simulink model "HF"  (Simulink 10.0)
settings: Solver=ode3  StartTime=0.0  StopTime=8  FixedStep=Tsim  RelTol=1e-3  EnableMultiTasking=on
InitFcn:
  | Tsim=2e-7;
values from neighbouring files (symbols this model uses):
  Flux = 0.00529276    [Hall_HFI_FOC_Data.sldd]
undefined symbols (not defined in the file or in its folder): DiscIntNeverNeededParam, sigbuilder_block
libraries: powerlib x10, powerlib_meascontrol x4, powerlib_extras x1, simulink_extras x1
settings Model: Creator=Administrator  LastModifiedBy=Administrator  SimulationMode=accelerator
settings DataIOCC: LimitDataPoints=on  SaveFormat=StructureWithTime
settings OptimizationCC: EfficientMapNaN2IntZero=off
settings DebuggingCC: UnderspecifiedInitializationDetection=Simplified  MergeDetectMultiDrivingBlocksExec=error
settings HardwareCC: ProdBitPerPointer=64  ProdLargestAtomicFloat=Float  ProdIntDivRoundTo=Zero  ProdEndianess=LittleEndian  ProdHWDeviceType=Specified  TargetBitPerPointer=64  TargetBitPerSizeT=64  TargetBitPerPtrDiffT=64  TargetLongLongMode=on  TargetIntDivRoundTo=Zero  TargetEndianess=LittleEndian  TargetWordSize=64  TargetHWDeviceType=MATLAB Host  ProdEqTarget=off
settings CodeAppCC: MaxIdLength=128
settings GRTTargetCC: GeneratePreprocessorConditionals=Disable all
settings ConfigComp: CovExternalEMLEnable=off
settings SimscapeCC: SimscapeNormalizeSystem=off

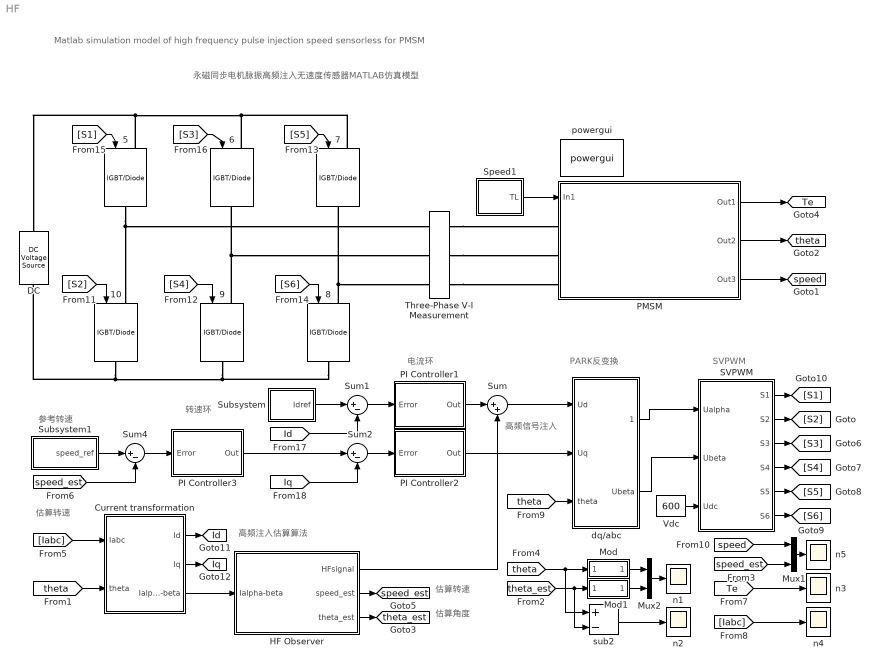
== system HF ==
  note: 转速环
  note: 永磁同步电机脉振高频注入无速度传感器MATLAB仿真模型
  note: Matlab simulation model of high frequency pulse injection speed sensorless for PMSM
  note: 电流环
  note: PARK反变换
  note: SVPWM
  note: 参考转速
  note: 估算转速
  note: 高频信号注入
  note: 估算转速
  note: 估算角度
  note: 高频注入估算算法
  {5..10} (6 alike) : powerlib/Power Electronics/IGBT//Diode  Ron=1e-3  Rs=5000  Cs=inf  Measurements=off
      settings: SourceProductName=Simscape Electrical
  Current transformation : Subsystem
  "DC " : powerlib/Electrical Sources/DC Voltage Source  Amplitude=600  Measurements=None
      settings: SourceProductName=Simscape Electrical
  HF Observer : Subsystem
  Mod : Subsystem
  Mod1 : Subsystem
  Mux1 : Mux  Inputs=2
  Mux2 : Mux  Inputs=2
  PI Controller1 : Subsystem  DialogController=POWERSYS.PowerSysDialog  mask(Discrete PI Controller){Kp=19.8, Ki=4550, Par_Limits=[346.4 -346.4], Init=0, Ts=1e-4}
      mask prompts: Kp "Proportional gain (Kp):"; Ki "Integral gain (Ki):"; Par_Limits "Output limits: [ Upper   Lower ]"; Init "Output initial value:"; Ts "Sample time:"
      mask help: This block implements a discrete PI controller.
      mask init:
      | UpperLimit=Par_Limits(1);
      | LowerLimit=Par_Limits(2);
      | power_initmask();
      mask Help: This block is part of a subset of blocks in the Extras library that does not have documentation associated with it, other than the block mask description.
      mask Display: disp('PI');
  PI Controller2 : Subsystem  DialogController=POWERSYS.PowerSysDialog  mask(Discrete PI Controller){Kp=19.9, Ki=4550, Par_Limits=[346.4 -346.4], Init=0, Ts=1e-4}
      mask prompts: Kp "Proportional gain (Kp):"; Ki "Integral gain (Ki):"; Par_Limits "Output limits: [ Upper   Lower ]"; Init "Output initial value:"; Ts "Sample time:"
      mask help: This block implements a discrete PI controller.
      mask init:
      | UpperLimit=Par_Limits(1);
      | LowerLimit=Par_Limits(2);
      | power_initmask();
      mask Help: This block is part of a subset of blocks in the Extras library that does not have documentation associated with it, other than the block mask description.
      mask Display: disp('PI');
  PI Controller3 : Subsystem  DialogController=POWERSYS.PowerSysDialog  mask(Discrete PI Controller){Kp=5, Ki=60, Par_Limits=[10 -10], Init=0, Ts=1e-4}
      mask prompts: Kp "Proportional gain (Kp):"; Ki "Integral gain (Ki):"; Par_Limits "Output limits: [ Upper   Lower ]"; Init "Output initial value:"; Ts "Sample time:"
      mask help: This block implements a discrete PI controller.
      mask init:
      | UpperLimit=Par_Limits(1);
      | LowerLimit=Par_Limits(2);
      | power_initmask();
      mask Help: This block is part of a subset of blocks in the Extras library that does not have documentation associated with it, other than the block mask description.
      mask Display: disp('PI');
  PMSM : Subsystem
      mask Display: image('PMSM.jpg');
  SVPWM : Subsystem  mask(Seven - sects SVPWM generator){fpwm=10e3, Ts=2e-7}
      mask prompts: fpwm "PWM frequency fpwm (Hz):"; Ts "Sample time Ts (s):"
      mask help: This block implements a space vector PWM.
  Speed1 : Subsystem  Tag=STV Subsys  LoadFcn=sigbuilder_block('load');  StartFcn=sigbuilder_block('start');  StopFcn=sigbuilder_block('stop');  ClipboardFcn=sigbuilder_block('clipboard');  mask(Sigbuilder block){tuvar=[0:10]}
      mask help: Simulink:masks:SigbuilderBlock_MD
      mask init:
      | if ~strcmp(get_param(bdroot(gcbh),'SimulationStatus'),'stopped') tuvar = sigbuilder_block('maskInit'); end
      settings: CopyFcn=sigbuilder_block('copy');  DeleteFcn=sigbuilder_block('delete');  ModelCloseFcn=sigbuilder_block('modelClose');  PreSaveFcn=sigbuilder_block('preSave');  PauseFcn=sigbuilder_block('pause');  ContinueFcn=sigbuilder_block('continue');  NameChangeFcn=sigbuilder_block('namechange');  OpenFcn=sigbuilder_block('open',[6 21.75 1012.5 490.5 ]);  CloseFcn=sigbuilder_block('close');
      mask Display: plot(0, 0, 100, 100,[2, 2, 32, 32, 2], [68, 8, 8, 68, 68],[32, 2], [38, 38], [32, 19, 2],[53, 60, 44], [32, 17, 17, 2],[16, 16, 31, 31]);txt = getActiveGroup(gcbh);text(2, 100, txt,'verticalAlignment', 'top');
  Subsystem : Subsystem
  Subsystem1 : Subsystem
  Sum : Sum  Inputs=|++
  Sum1 : Sum  Inputs=|+-
  Sum2 : Sum  Inputs=|+-
  Sum4 : Sum  Inputs=|+-
  Three-Phase V-I Measurement : powerlib/Measurements/Three-Phase V-I Measurement  VoltageMeasurement=phase-to-phase  SetLabelV=on  LabelV=Vabc  Vpu=off  VpuLL=off  CurrentMeasurement=yes  SetLabelI=on  LabelI=Iabc  Ipu=off  Pbase=100e6  Vbase=500e3  OutputType=Complex  PhasorSimulation=off  PSBequivalent=0
      settings: SourceProductName=Simscape Electrical
  Vdc : Constant  Value=600
  dq/abc : Subsystem
  n{1..5} (5 alike) : Scope
  powergui : powerlib/powergui  Priority=1  SimulationMode=Discrete  SampleTime=0.002*1e-4  frequency=60  Iterations=50  frequencyindice=0  Pbase=100e6  ErrMax=1e-4  UnitsV=kV  UnitsW=MW  buscounter=0  FunctionMessages=off  echomessages=off  EnableUseOfTLC=off  CurrentSourceSwitches=off  DisableSnubberDevices=off  DisableRonSwitches=off  DisableVfSwitches=off  DisplayEquations=off  AutomaticDiscreteSolvers=off  SolverType=Tustin/Backward Euler (TBE)  Interpol=off  ExternalGateDelay=off  methode=off  Ts=10  x0status=blocks  SPID=off  SwTol=0  HookPort=off  NonlinearTolerance=1e-4  nMaxIteration=100  ContinueOnMaxIteration=off  RestoreLinks=warning  ResistiveCurrentMeasurement=off  Frange=[0:2:500]  Ylog=off  Xlog=on  ShowGrid=off  save=off  variable=ZData  structure=0  ZoomFFT=off  StartTime=0.0  cycles=1  DisplayStyle=1  fundamental=60  FreqAxis=off  MaxFrequency=1000  frequencyindicesteady=1  RmsSteady=1  display=off
      settings: SourceProductName=Simscape Electrical
  sub2 : Sum  Inputs=+-
  tag scope: Id=global, Iq=global, Te=global, speed=global, speed_est=global, theta=global, theta_est=global
  wires:
  dq/abc/1(Ualpha) -> SVPWM/1(Ualpha)
  PI Controller3/1(Out) -> Sum2/1
  HF Observer/3(theta_est) -> [theta_est]
  HF Observer/1(HFsignal) -> Sum/2
  PI Controller1/1(Out) -> Sum/1
  Vdc/1 -> SVPWM/3(Udc)
  Sum1/1 -> PI Controller1/1(Error)
  Sum2/1 -> PI Controller2/1(Error)
  Sum4/1 -> PI Controller3/1(Error)
  Mux2/1 -> n1/1
  Mod/1(Out1) -> Mux2/1
  Mod1/1(Out1) -> Mux2/2
  [theta] -> Current transformation/2(theta)
  [theta] -> dq/abc/3(theta)
  [theta_est] -> sub2/2, Mod1/1(In1)
  [theta] -> sub2/1, Mod/1(In1)
  sub2/1 -> n2/1
  PI Controller2/1(Out) -> dq/abc/2(Uq)
  Sum/1 -> dq/abc/1(Ud)
  dq/abc/2(Ubeta) -> SVPWM/2(Ubeta)
  [S1] -> 5/1
  [S2] -> 10/1
  [S3] -> 6/1
  [S4] -> 9/1
  [S5] -> 7/1
  [S6] -> 8/1
  SVPWM/1(S1) -> [S1]
  SVPWM/2(S2) -> [S2]
  SVPWM/3(S3) -> [S3]
  SVPWM/4(S4) -> [S4]
  SVPWM/5(S5) -> [S5]
  SVPWM/6(S6) -> [S6]
  [Iabc] -> Current transformation/1(Iabc)
  Speed1/1(TL) -> PMSM/1(In1)
  PMSM/1(Out1) -> [Te]
  PMSM/2(Out2) -> [theta]
  PMSM/3(Out3) -> [speed]
  [Te] -> n3/1
  [Iabc] -> n4/1
  Current transformation/3(Ialpha-beta) -> HF Observer/1(Ialpha-beta)
  HF Observer/2(speed_est) -> [speed_est]
  [speed_est] -> Sum4/2
  Mux1/1 -> n5/1
  [speed_est] -> Mux1/2
  [speed] -> Mux1/1
  Current transformation/1(Id) -> [Id]
  Current transformation/2(Iq) -> [Iq]
  [Id] -> Sum1/2
  [Iq] -> Sum2/2
  Subsystem1/1(speed_ref) -> Sum4/1
  Subsystem/1(Idref) -> Sum1/1
  connections:
  10/RConn1 -- "DC "/LConn1 -- 8/RConn1 -- 9/RConn1
  5/RConn1 -- Three-Phase V-I Measurement/LConn1 -- 10/LConn1
  9/LConn1 -- Three-Phase V-I Measurement/LConn2 -- 6/RConn1
  8/LConn1 -- Three-Phase V-I Measurement/LConn3 -- 7/RConn1
  5/LConn1 -- "DC "/RConn1 -- 6/LConn1 -- 7/LConn1
  Three-Phase V-I Measurement/RConn1 -- PMSM/LConn1
  Three-Phase V-I Measurement/RConn2 -- PMSM/LConn2
  Three-Phase V-I Measurement/RConn3 -- PMSM/LConn3

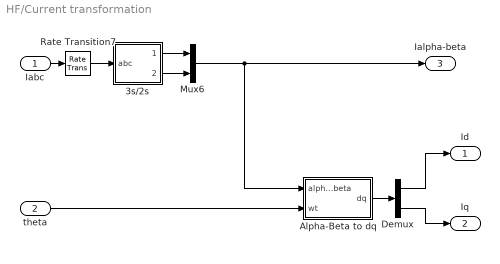
== system HF/Current transformation ==
  Iabc : Inport
  theta : Inport  Port=2
  3s/2s : Subsystem
  Alpha-Beta to dq : Subsystem
      mask Display:
      | plot([0 1], [0,1])
      | port_label('input', 1, '\alpha\beta','texmode','on')
      | port_label('input', 2, 'wt')
      | port_label('output', 1, 'dq')
  Demux : Demux  Outputs=2
  Mux6 : Mux  Inputs=2
  Rate Transition7 : RateTransition
  Id : Outport
  Iq : Outport  Port=2
  Ialpha-beta : Outport  Port=3
  wires:
  Iabc/1 -> Rate Transition7/1
  3s/2s/1(alpha) -> Mux6/1
  3s/2s/2(beta) -> Mux6/2
  Mux6/1 -> Ialpha-beta/1, Alpha-Beta to dq/1(alpha_beta)
  theta/1 -> Alpha-Beta to dq/2(wt)
  Alpha-Beta to dq/1(dq) -> Demux/1
  Demux/1 -> Id/1
  Demux/2 -> Iq/1
  Rate Transition7/1 -> 3s/2s/1(abc)

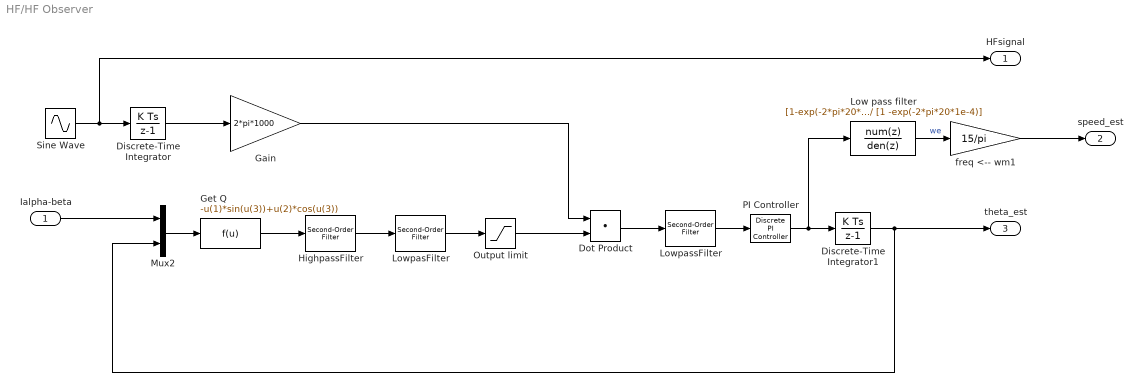
== system HF/HF Observer ==
  Ialpha-beta : Inport
  Discrete-Time Integrator : DiscreteIntegrator  SampleTime=-1  ICPrevOutput=DiscIntNeverNeededParam  ICPrevScaledInput=DiscIntNeverNeededParam
  Discrete-Time Integrator1 : DiscreteIntegrator  SampleTime=-1  ICPrevOutput=DiscIntNeverNeededParam  ICPrevScaledInput=DiscIntNeverNeededParam
  Dot Product : DotProduct  InputSameDT=on  OutDataTypeStr=Inherit: Inherit via internal rule
  Gain : Gain  Gain=2*pi*1000
  Get Q : Fcn  Expr=-u(1)*sin(u(3))+u(2)*cos(u(3))
  HighpassFilter : powerlib_meascontrol/Filters/Second-Order Filter  FilterType=Highpass  Fo=1000 - 100/2  Zeta=0.3  Ts=1e-4  Initialize=off  Vac_Init="[0,  0,  60]"  Vdc_Init=0  PlotResponse=off  FreqRange=[0, 10000, 1]
      settings: SourceProductName=Simscape Electrical  SourceProductBaseCode=PS
  Low pass filter : DiscreteTransferFcn  Numerator=[1-exp(-2*pi*20*1e-4)]  Denominator=[1 -exp(-2*pi*20*1e-4)]  SampleTime=1e-4
  LowpasFilter : powerlib_meascontrol/Filters/Second-Order Filter  FilterType=Lowpass  Fo=1000 + 100/2  Zeta=0.3  Ts=1e-4  Initialize=off  Vac_Init="[0,  0,  60]"  Vdc_Init=0  PlotResponse=off  FreqRange=[0, 5000, 1]
      settings: SourceProductName=Simscape Electrical  SourceProductBaseCode=PS
  LowpassFilter : powerlib_meascontrol/Filters/Second-Order Filter  FilterType=Lowpass  Fo=100  Zeta=0.707  Ts=1e-4  Initialize=off  Vac_Init="[0,  0,  60]"  Vdc_Init=0  PlotResponse=off  FreqRange=[0, 500, 1]
      settings: SourceProductName=Simscape Electrical  SourceProductBaseCode=PS
  Mux2 : Mux  Inputs=2
  Output limit : Saturate
  PI Controller : powerlib_extras/Discrete  Control Blocks/Discrete PI Controller  Kp=5  Ki=50  Par_Limits=[100*2*pi -100*2*pi]  Init=0  Ts=1e-4
      settings: SourceProductName=Simscape Electrical
  Sine Wave : Sin  Amplitude=20  Frequency=2*pi*1000  Phase=pi/2  SampleTime=1e-4
  freq <-- wm1 : Gain  Gain=15/pi
  HFsignal : Outport
  speed_est : Outport  Port=2
  theta_est : Outport  Port=3
  wires:
  Ialpha-beta/1 -> Mux2/1
  Get Q/1 -> HighpassFilter/1
  HighpassFilter/1 -> LowpasFilter/1
  Sine Wave/1 -> HFsignal/1, Discrete-Time Integrator/1
  Discrete-Time Integrator/1 -> Gain/1
  Gain/1 -> Dot Product/1
  Dot Product/1 -> LowpassFilter/1
  LowpassFilter/1 -> PI Controller/1
  PI Controller/1 -> Low pass filter/1, Discrete-Time Integrator1/1
  Output limit/1 -> Dot Product/2
  LowpasFilter/1 -> Output limit/1
  Discrete-Time Integrator1/1 -> theta_est/1, Mux2/2
  Mux2/1 -> Get Q/1
  Low pass filter/1 -> freq <-- wm1/1  "we"
  freq <-- wm1/1 -> speed_est/1

== system HF/Mod ==
  In1 : Inport
  Constant1 : Constant  Value=2*pi
  Math Function : Math  Operator=mod  SaturateOnIntegerOverflow=on
  Out1 : Outport
  wires:
  Constant1/1 -> Math Function/2
  Math Function/1 -> Out1/1
  In1/1 -> Math Function/1

== system HF/Mod1 ==
  In1 : Inport
  Constant1 : Constant  Value=2*pi
  Math Function : Math  Operator=mod  SaturateOnIntegerOverflow=on
  Out1 : Outport
  wires:
  In1/1 -> Math Function/1
  Math Function/1 -> Out1/1
  Constant1/1 -> Math Function/2

== system HF/PI Controller1 ==
  Error : Inport  SampleTime=Ts
  Discrete-Time Integrator : DiscreteIntegrator  InitialCondition=Init  SampleTime=Ts  LimitOutput=on  UpperSaturationLimit=UpperLimit  LowerSaturationLimit=LowerLimit  ICPrevOutput=DiscIntNeverNeededParam  ICPrevScaledInput=DiscIntNeverNeededParam
  Kp4 : Gain  Gain=Kp  SampleTime=Ts  SaturateOnIntegerOverflow=on  OutDataTypeStr=Inherit: Same as input  ParamDataTypeStr=Inherit: Same as input
  Kp5 : Gain  Gain=Ki  SampleTime=Ts  SaturateOnIntegerOverflow=on  OutDataTypeStr=Inherit: Same as input  ParamDataTypeStr=Inherit: Same as input
  Saturation2 : Saturate  UpperLimit=UpperLimit  LowerLimit=LowerLimit  SampleTime=Ts
  Sum6 : Sum  SampleTime=Ts  SaturateOnIntegerOverflow=on  InputSameDT=on  OutDataTypeStr=Inherit: Same as first input
  Zero-Order Hold : ZeroOrderHold  SampleTime=Ts
  Out : Outport  SampleTime=Ts  InitialOutput=0
  wires:
  Zero-Order Hold/1 -> Sum6/1
  Discrete-Time Integrator/1 -> Sum6/2
  Kp4/1 -> Zero-Order Hold/1
  Kp5/1 -> Discrete-Time Integrator/1
  Sum6/1 -> Saturation2/1
  Error/1 -> Kp5/1, Kp4/1
  Saturation2/1 -> Out/1

== system HF/PI Controller2 ==
  Error : Inport  SampleTime=Ts
  Discrete-Time Integrator : DiscreteIntegrator  InitialCondition=Init  SampleTime=Ts  LimitOutput=on  UpperSaturationLimit=UpperLimit  LowerSaturationLimit=LowerLimit  ICPrevOutput=DiscIntNeverNeededParam  ICPrevScaledInput=DiscIntNeverNeededParam
  Kp4 : Gain  Gain=Kp  SampleTime=Ts  SaturateOnIntegerOverflow=on  OutDataTypeStr=Inherit: Same as input  ParamDataTypeStr=Inherit: Same as input
  Kp5 : Gain  Gain=Ki  SampleTime=Ts  SaturateOnIntegerOverflow=on  OutDataTypeStr=Inherit: Same as input  ParamDataTypeStr=Inherit: Same as input
  Saturation2 : Saturate  UpperLimit=UpperLimit  LowerLimit=LowerLimit  SampleTime=Ts
  Sum6 : Sum  SampleTime=Ts  SaturateOnIntegerOverflow=on  InputSameDT=on  OutDataTypeStr=Inherit: Same as first input
  Zero-Order Hold : ZeroOrderHold  SampleTime=Ts
  Out : Outport  SampleTime=Ts  InitialOutput=0
  wires:
  Zero-Order Hold/1 -> Sum6/1
  Discrete-Time Integrator/1 -> Sum6/2
  Kp4/1 -> Zero-Order Hold/1
  Kp5/1 -> Discrete-Time Integrator/1
  Sum6/1 -> Saturation2/1
  Error/1 -> Kp5/1, Kp4/1
  Saturation2/1 -> Out/1

== system HF/PI Controller3 ==
  Error : Inport  SampleTime=Ts
  Discrete-Time Integrator : DiscreteIntegrator  InitialCondition=Init  SampleTime=Ts  LimitOutput=on  UpperSaturationLimit=UpperLimit  LowerSaturationLimit=LowerLimit  ICPrevOutput=DiscIntNeverNeededParam  ICPrevScaledInput=DiscIntNeverNeededParam
  Iq_calcu_limit : Subsystem
  Kp4 : Gain  Gain=Kp  SampleTime=Ts  SaturateOnIntegerOverflow=on  OutDataTypeStr=Inherit: Same as input  ParamDataTypeStr=Inherit: Same as input
  Kp5 : Gain  Gain=Ki  SampleTime=Ts  SaturateOnIntegerOverflow=on  OutDataTypeStr=Inherit: Same as input  ParamDataTypeStr=Inherit: Same as input
  Saturation2 : Saturate  UpperLimit=UpperLimit  LowerLimit=LowerLimit  SampleTime=Ts
  Sum6 : Sum  SampleTime=Ts  SaturateOnIntegerOverflow=on  InputSameDT=on  OutDataTypeStr=Inherit: Same as first input
  Zero-Order Hold : ZeroOrderHold  SampleTime=Ts
  freq <-- wm1 : Gain  Gain=1/30
  Out : Outport  SampleTime=Ts  InitialOutput=0
  wires:
  Zero-Order Hold/1 -> Sum6/1
  Discrete-Time Integrator/1 -> Sum6/2
  Kp4/1 -> Zero-Order Hold/1
  Kp5/1 -> Discrete-Time Integrator/1
  Sum6/1 -> Saturation2/1
  Saturation2/1 -> Iq_calcu_limit/1(Te_ref)
  Iq_calcu_limit/1(Iq_ref) -> Out/1
  Error/1 -> freq <-- wm1/1
  freq <-- wm1/1 -> Kp4/1, Kp5/1

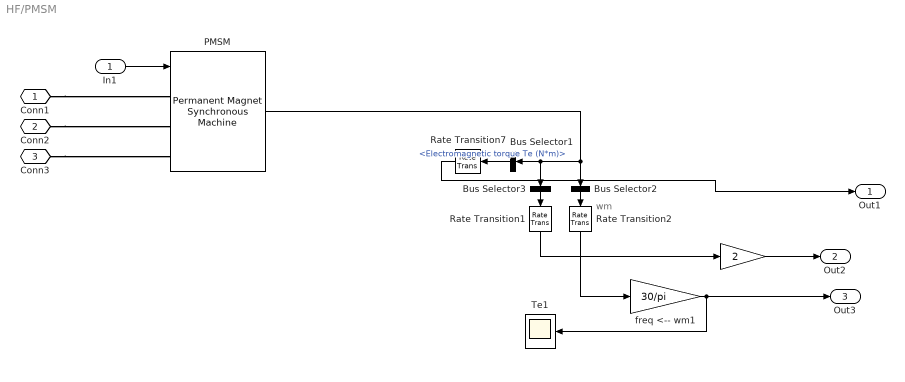
== system HF/PMSM ==
  note: wm
  In1 : Inport
  " " : Gain  Gain=2  SaturateOnIntegerOverflow=on  OutDataTypeStr=Inherit: Same as input  ParamDataTypeStr=Inherit: Same as input
  Bus Selector1 : BusSelector  OutputSignals=Electromagnetic torque Te (N*m)
  Bus Selector2 : BusSelector  OutputSignals=Rotor speed wm (rad/s)  OutputAsBus=on
  Bus Selector3 : BusSelector  OutputSignals=Rotor angle thetam (rad)  OutputAsBus=on
  PMSM : powerlib/Machines/Permanent Magnet Synchronous Machine  NbPhases=3  FluxDistribution=Sinusoidal  RotorType=Salient-pole  MechanicalLoad=Torque Tm  PresetModel=No  ShowDetailedParameters=on  MeasurementBus=off  Resistance=0.91  Inductance=8.5e-3  dqInductances=[3.96e-3,7.96e-3]  La=Ls  MachineConstant=Flux linkage established by magnets (V.s)  Flux=0.446  VoltageCst=161.7909  TorqueCst=1.338  Flat=120  Mechanical=[0.074 0.008 2 0]  PolePairs=4  InitialConditions=[0,0, 0,0]  InitialConditions5ph=[0 0 0 0 0 0]  RefAngle=Aligned with phase A axis (original Park)  IterativeDiscreteModel=Trapezoidal non iterative  TsBlock=-1  TsPowergui=0
  Rate Transition1 : RateTransition  OutPortSampleTime=1e-4
  Rate Transition2 : RateTransition  OutPortSampleTime=1e-4
  Rate Transition7 : RateTransition
  Te1 : Scope
  freq <-- wm1 : Gain  Gain=30/pi
  Conn1 : PMIOPort  Side=Left
  Conn2 : PMIOPort  Port=2  Side=Left
  Conn3 : PMIOPort  Port=3  Side=Left
  Out1 : Outport
  Out2 : Outport  Port=2
  Out3 : Outport  Port=3
  wires:
  freq <-- wm1/1 -> Out3/1, Te1/1
  " "/1 -> Out2/1
  In1/1 -> PMSM/1
  Bus Selector1/1 -> Rate Transition7/1  "<Electromagnetic torque Te (N*m)>"
  Bus Selector2/1 -> Rate Transition2/1
  PMSM/1 -> Bus Selector2/1, Bus Selector1/1, Bus Selector3/1
  Rate Transition7/1 -> Out1/1
  Bus Selector3/1 -> Rate Transition1/1
  Rate Transition2/1 -> freq <-- wm1/1
  Rate Transition1/1 -> " "/1
  connections:
  Conn2/RConn1 -- PMSM/LConn2
  Conn3/RConn1 -- PMSM/LConn3
  Conn1/RConn1 -- PMSM/LConn1

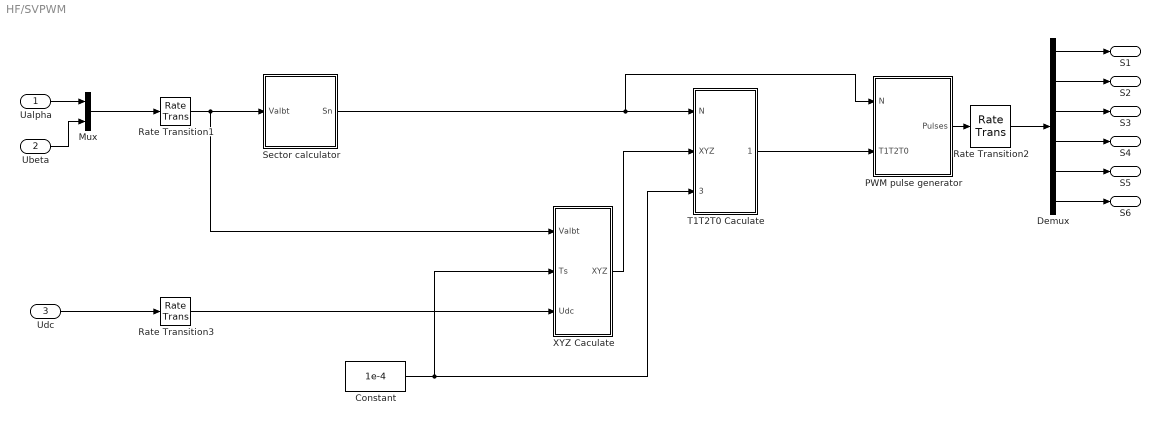
== system HF/SVPWM ==
  Ualpha : Inport
  Ubeta : Inport  Port=2
  Udc : Inport  Port=3
  Constant : Constant  Value=1e-4
  Demux : Demux  Outputs=6
  Mux : Mux  Inputs=2
  PWM pulse generator : Subsystem
  Rate Transition1 : RateTransition  OutPortSampleTimeOpt=Inherit
  Rate Transition2 : RateTransition
  Rate Transition3 : RateTransition  OutPortSampleTimeOpt=Inherit
  Sector calculator : Subsystem
  T1T2T0 Caculate : Subsystem
  XYZ Caculate : Subsystem
  S1 : Outport
  S2 : Outport  Port=2
  S3 : Outport  Port=3
  S4 : Outport  Port=4
  S5 : Outport  Port=5
  S6 : Outport  Port=6
  wires:
  XYZ Caculate/1(XYZ) -> T1T2T0 Caculate/2(XYZ)
  Rate Transition3/1 -> XYZ Caculate/3(Udc)
  Constant/1 -> XYZ Caculate/2(Ts), T1T2T0 Caculate/3(Tpwm)
  PWM pulse generator/1(Pulses) -> Rate Transition2/1
  Sector calculator/1(Sn) -> PWM pulse generator/1(N), T1T2T0 Caculate/1(N)
  Rate Transition1/1 -> Sector calculator/1(Valbt), XYZ Caculate/1(Valbt)
  Udc/1 -> Rate Transition3/1
  T1T2T0 Caculate/1(T1T2T0) -> PWM pulse generator/2(T1T2T0)
  Ualpha/1 -> Mux/1
  Ubeta/1 -> Mux/2
  Mux/1 -> Rate Transition1/1
  Rate Transition2/1 -> Demux/1
  Demux/1 -> S1/1
  Demux/2 -> S2/1
  Demux/3 -> S3/1
  Demux/4 -> S4/1
  Demux/5 -> S5/1
  Demux/6 -> S6/1

== system HF/Speed1 ==
  Demux : Demux  Tag=STV Demux  Outputs=1
  FromWs : FromWorkspace  Tag=STV FromWs  VariableName=tuvar  SampleTime=0  SigBuilderData=DataTag0  VnvData=DataTag1
      SigBuilderData=|
      | common.afterFinalStr = 'Extrapolate'
      | common.sampleTime = 0
      | dataSet.timeRange = [0 10]
      | dataSet.name = '负载转矩'
      | sbobj.Groups.Name = '负载转矩'
      | sbobj.Groups.Signals.Name = 'TL'
      | sbobj.Groups.Signals.XData = [0 5 5 6 6 10]
      | sbobj.Groups.Signals.YData = [0 0 6 6 0 0]
  TL : Outport  Tag=STV Outport
  wires:
  FromWs/1 -> Demux/1
  Demux/1 -> TL/1

== system HF/Subsystem ==
  id : Constant  Value=0
  Idref : Outport
  wires:
  id/1 -> Idref/1

== system HF/Subsystem1 ==
  Rate Transition3 : RateTransition  OutPortSampleTime=1e-4
  Speed2 : Subsystem  Tag=STV Subsys  LoadFcn=sigbuilder_block('load');  StartFcn=sigbuilder_block('start');  StopFcn=sigbuilder_block('stop');  ClipboardFcn=sigbuilder_block('clipboard');  mask(Sigbuilder block){tuvar=[0:10]}
      mask help: Simulink:masks:SigbuilderBlock_MD
      mask init:
      | if ~strcmp(get_param(bdroot(gcbh),'SimulationStatus'),'stopped') tuvar = sigbuilder_block('maskInit'); end
      settings: CopyFcn=sigbuilder_block('copy');  DeleteFcn=sigbuilder_block('delete');  ModelCloseFcn=sigbuilder_block('modelClose');  PreSaveFcn=sigbuilder_block('preSave');  PauseFcn=sigbuilder_block('pause');  ContinueFcn=sigbuilder_block('continue');  NameChangeFcn=sigbuilder_block('namechange');  OpenFcn=sigbuilder_block('open',[6 21.75 1012.5 490.5 ]);  CloseFcn=sigbuilder_block('close');
      mask Display: plot(0, 0, 100, 100,[2, 2, 32, 32, 2], [68, 8, 8, 68, 68],[32, 2], [38, 38], [32, 19, 2],[53, 60, 44], [32, 17, 17, 2],[16, 16, 31, 31]);txt = getActiveGroup(gcbh);text(2, 100, txt,'verticalAlignment', 'top');
  speed_ref : Outport
  wires:
  Speed2/1(Speed) -> Rate Transition3/1
  Rate Transition3/1 -> speed_ref/1

== system HF/dq/abc ==
  Ud : Inport
  Uq : Inport  Port=2
  theta : Inport  Port=3
  Fcn : Fcn  Expr=u(1)*u(4)-u(2)*u(3)
  Fcn1 : Fcn  Expr=u(1)*u(3)+u(2)*u(4)
  Mux : Mux
  Trigonometric Function : Trigonometry
  Trigonometric Function1 : Trigonometry  Operator=cos
  Ualpha : Outport
  Ubeta : Outport  Port=2
  wires:
  theta/1 -> Trigonometric Function1/1, Trigonometric Function/1
  Trigonometric Function1/1 -> Mux/4
  Trigonometric Function/1 -> Mux/3
  Ud/1 -> Mux/1
  Mux/1 -> Fcn1/1, Fcn/1
  Fcn/1 -> Ualpha/1
  Uq/1 -> Mux/2
  Fcn1/1 -> Ubeta/1

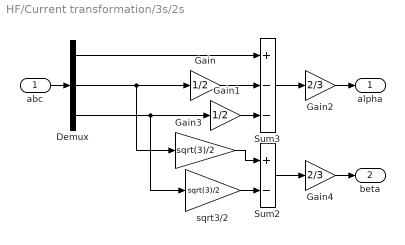
== system HF/Current transformation/3s/2s ==
  abc : Inport
  Demux : Demux  Outputs=3
  Gain : Gain  Gain=1/2  SaturateOnIntegerOverflow=on  OutDataTypeStr=Inherit: Same as input  ParamDataTypeStr=Inherit: Same as input
  Gain1 : Gain  Gain=1/2  SaturateOnIntegerOverflow=on  OutDataTypeStr=Inherit: Same as input  ParamDataTypeStr=Inherit: Same as input
  Gain2 : Gain  Gain=2/3  SaturateOnIntegerOverflow=on  OutDataTypeStr=Inherit: Same as input  ParamDataTypeStr=Inherit: Same as input
  Gain3 : Gain  Gain=sqrt(3)/2  SaturateOnIntegerOverflow=on  OutDataTypeStr=Inherit: Same as input  ParamDataTypeStr=Inherit: Same as input
  Gain4 : Gain  Gain=2/3  SaturateOnIntegerOverflow=on  OutDataTypeStr=Inherit: Same as input  ParamDataTypeStr=Inherit: Same as input
  Sum2 : Sum  Inputs=+-  SaturateOnIntegerOverflow=on  InputSameDT=on  OutDataTypeStr=Inherit: Same as first input
  Sum3 : Sum  Inputs=+--  SaturateOnIntegerOverflow=on  InputSameDT=on  OutDataTypeStr=Inherit: Same as first input
  sqrt3/2 : Gain  Gain=sqrt(3)/2  SaturateOnIntegerOverflow=on  OutDataTypeStr=Inherit: Same as input  ParamDataTypeStr=Inherit: Same as input
  alpha : Outport
  beta : Outport  Port=2
  wires:
  Sum2/1 -> Gain4/1
  Gain2/1 -> alpha/1
  abc/1 -> Demux/1
  Demux/1 -> Sum3/1
  Demux/2 -> Gain/1, Gain3/1
  Gain1/1 -> Sum3/3
  Gain/1 -> Sum3/2
  Demux/3 -> Gain1/1, sqrt3/2/1
  Gain3/1 -> Sum2/1
  sqrt3/2/1 -> Sum2/2
  Gain4/1 -> beta/1
  Sum3/1 -> Gain2/1

== system HF/Current transformation/Alpha-Beta to dq ==
  note: d = al*cos(wt) + be*sin(wt)
  note: q = -al*sin(wt) + be*cos(wt)
  note: [  al
      |     be  ]
  note: [ d
      |    q ]
  note: *
  note: =
  note: [  cos(wt)   sin(wt)
      |    -sin(wt)    cos(wt)   ]
  alpha_beta : Inport  PortDimensions=2
  wt : Inport  Port=2  PortDimensions=1
  Fcn : Fcn  Expr=u[1]*cos(u[3]) + u[2]*sin(u[3])
  Fcn1 : Fcn  Expr=-u[1]*sin(u[3]) + u[2]*cos(u[3])
  Mux : Mux  Inputs=2
  Mux1 : Mux  Inputs=[2 1]
  Mux2 : Mux  Inputs=[2 1]
  dq : Outport  InitialOutput=[0,0]
  wires:
  Mux1/1 -> Fcn/1
  wt/1 -> Mux1/2, Mux2/2
  alpha_beta/1 -> Mux1/1, Mux2/1
  Mux2/1 -> Fcn1/1
  Fcn/1 -> Mux/1
  Fcn1/1 -> Mux/2
  Mux/1 -> dq/1

== system HF/PI Controller3/Iq_calcu_limit ==
  Te_ref : Inport
  Fcn : Fcn  Expr=(2/3)*u/2/0.446
  Output limit1 : Saturate  UpperLimit=11  LowerLimit=-11
  Iq_ref : Outport  InitialOutput=0
  wires:
  Te_ref/1 -> Fcn/1
  Fcn/1 -> Output limit1/1
  Output limit1/1 -> Iq_ref/1

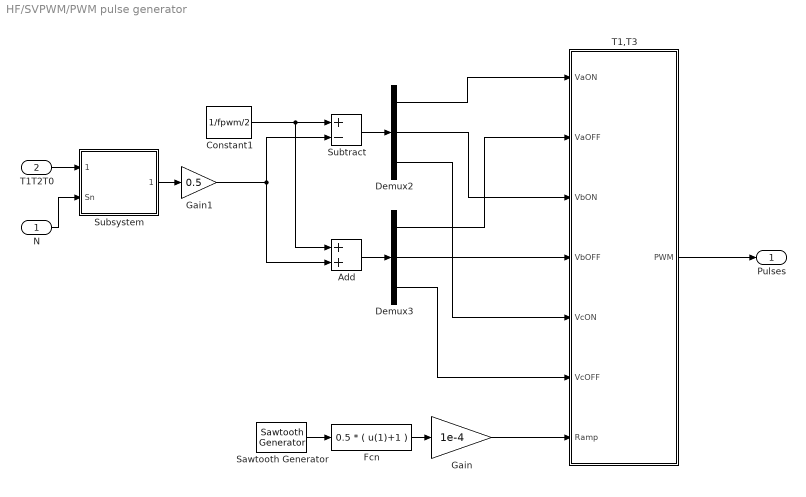
== system HF/SVPWM/PWM pulse generator ==
  N : Inport
  T1T2T0 : Inport  Port=2
  Add : Sum
  Constant1 : Constant  Value=1/fpwm/2
  Demux2 : Demux  Outputs=3
  Demux3 : Demux  Outputs=3
  Fcn : Fcn  Expr=0.5 * ( u(1)+1 )
  Gain : Gain  Gain=1e-4
  Gain1 : Gain  Gain=0.5
  Sawtooth Generator : powerlib_meascontrol/Pulse & Signal Generators/Sawtooth Generator  Freq=fpwm  Phase=0  Ts=Ts
      settings: SourceProductName=Simscape Electrical
  Subsystem : Subsystem
  Subtract : Sum  Inputs=+-
  T1,T3 : Subsystem
  Pulses : Outport
  wires:
  Gain/1 -> T1,T3/7(Ramp)
  Fcn/1 -> Gain/1
  T1,T3/1(PWM) -> Pulses/1
  Sawtooth Generator/1 -> Fcn/1
  Demux3/3 -> T1,T3/6(VcOFF)
  Demux2/3 -> T1,T3/5(VcON)
  Demux3/2 -> T1,T3/4(VbOFF)
  Demux2/2 -> T1,T3/3(VbON)
  Demux3/1 -> T1,T3/2(VaOFF)
  Demux2/1 -> T1,T3/1(VaON)
  Add/1 -> Demux3/1
  Subtract/1 -> Demux2/1
  N/1 -> Subsystem/2(Sn)
  Constant1/1 -> Subtract/1, Add/1
  Gain1/1 -> Subtract/2, Add/2
  Subsystem/1(Tabc_on) -> Gain1/1
  T1T2T0/1 -> Subsystem/1(T1T2T0)

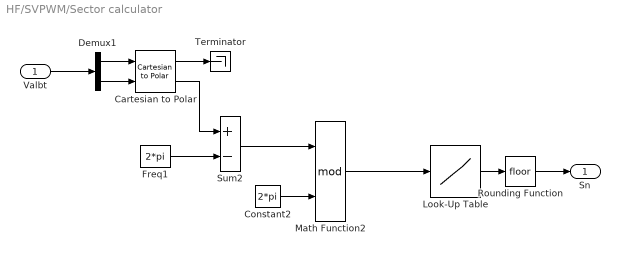
== system HF/SVPWM/Sector calculator ==
  Valbt : Inport
  Cartesian to Polar : simulink_extras/Transformations/Cartesian to Polar
      settings: SourceProductName=Simulink
  Constant2 : Constant  Value=2*pi
  Demux1 : Demux  Outputs=2
  Freq1 : Constant  Value=2*pi
  Look-Up Table : Lookup  InputValues=[0:pi/3:5*pi/3]  Table=[1:6]  SaturateOnIntegerOverflow=on
  Math Function2 : Math  Operator=mod  SaturateOnIntegerOverflow=on
  Rounding Function : Rounding
  Sum2 : Sum  Inputs=+-  SaturateOnIntegerOverflow=on  InputSameDT=on  OutDataTypeStr=Inherit: Same as first input
  Terminator : Terminator
  Sn : Outport
  wires:
  Math Function2/1 -> Look-Up Table/1
  Constant2/1 -> Math Function2/2
  Sum2/1 -> Math Function2/1
  Freq1/1 -> Sum2/2
  Look-Up Table/1 -> Rounding Function/1
  Rounding Function/1 -> Sn/1
  Cartesian to Polar/2 -> Sum2/1
  Cartesian to Polar/1 -> Terminator/1
  Demux1/2 -> Cartesian to Polar/2
  Demux1/1 -> Cartesian to Polar/1
  Valbt/1 -> Demux1/1

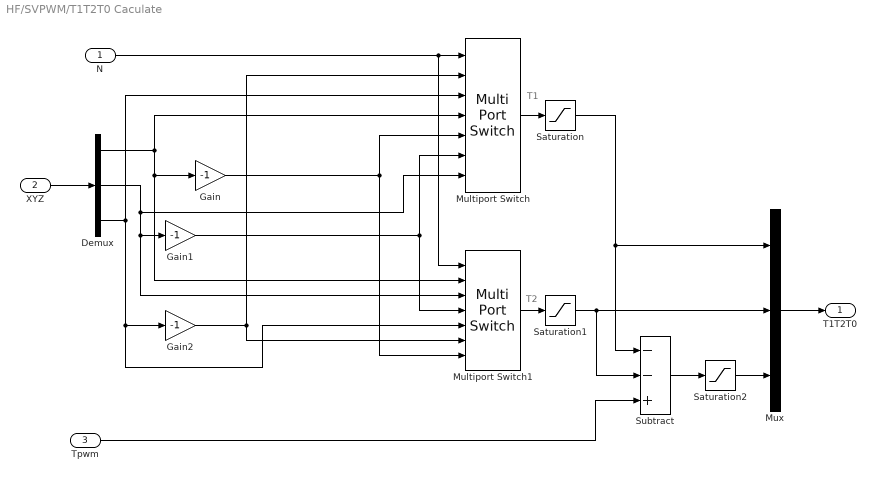
== system HF/SVPWM/T1T2T0 Caculate ==
  note: T2
  note: T1
  N : Inport
  XYZ : Inport  Port=2
  Tpwm : Inport  Port=3
  Demux : Demux  Outputs=3
  Gain : Gain  Gain=-1
  Gain1 : Gain  Gain=-1
  Gain2 : Gain  Gain=-1
  Multiport Switch : MultiPortSwitch  Inputs=6
  Multiport Switch1 : MultiPortSwitch  Inputs=6
  Mux : Mux  Inputs=3
  Saturation : Saturate  UpperLimit=1/fpwm  LowerLimit=0
  Saturation1 : Saturate  UpperLimit=1/fpwm  LowerLimit=0
  Saturation2 : Saturate  UpperLimit=1/fpwm  LowerLimit=0
  Subtract : Sum  Inputs=--+
  T1T2T0 : Outport
  wires:
  Mux/1 -> T1T2T0/1
  Tpwm/1 -> Subtract/3
  Subtract/1 -> Saturation2/1
  Gain/1 -> Multiport Switch1/7, Multiport Switch/5
  Gain1/1 -> Multiport Switch/6, Multiport Switch1/4
  Gain2/1 -> Multiport Switch1/6, Multiport Switch/2
  Demux/1 -> Multiport Switch1/2, Gain/1, Multiport Switch/4
  Demux/3 -> Multiport Switch/3, Gain2/1, Multiport Switch1/5
  Demux/2 -> Gain1/1, Multiport Switch1/3, Multiport Switch/7
  N/1 -> Multiport Switch/1, Multiport Switch1/1
  Multiport Switch1/1 -> Saturation1/1
  Multiport Switch/1 -> Saturation/1
  XYZ/1 -> Demux/1
  Saturation/1 -> Mux/1, Subtract/1
  Saturation1/1 -> Mux/2, Subtract/2
  Saturation2/1 -> Mux/3

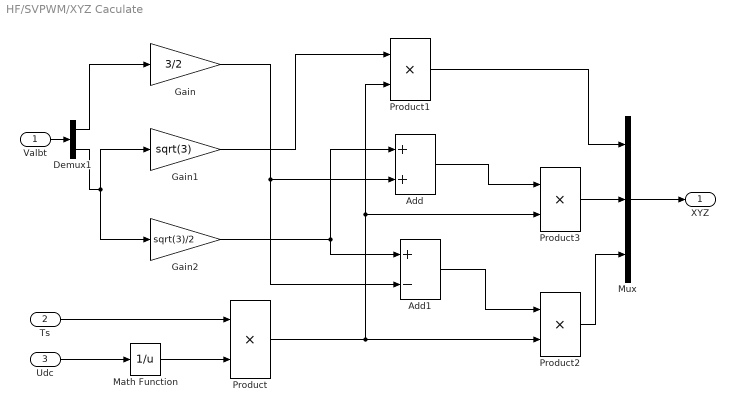
== system HF/SVPWM/XYZ Caculate ==
  Valbt : Inport
  Ts : Inport  Port=2
  Udc : Inport  Port=3
  Add : Sum
  Add1 : Sum  Inputs=+-
  Demux1 : Demux  Outputs=2
  Gain : Gain  Gain=3/2
  Gain1 : Gain  Gain=sqrt(3)
  Gain2 : Gain  Gain=sqrt(3)/2
  Math Function : Math  Operator=reciprocal  SaturateOnIntegerOverflow=on
  Mux : Mux  Inputs=3
  Product{,1..3} (4 alike) : Product  RndMeth=Zero
  XYZ : Outport
  wires:
  Valbt/1 -> Demux1/1
  Add/1 -> Product3/1
  Add1/1 -> Product2/1
  Gain2/1 -> Add1/1, Add/1
  Gain/1 -> Add/2, Add1/2
  Product/1 -> Product3/2, Product1/2, Product2/2
  Gain1/1 -> Product1/1
  Ts/1 -> Product/1
  Math Function/1 -> Product/2
  Udc/1 -> Math Function/1
  Demux1/2 -> Gain1/1, Gain2/1
  Demux1/1 -> Gain/1
  Product2/1 -> Mux/3
  Product3/1 -> Mux/2
  Product1/1 -> Mux/1
  Mux/1 -> XYZ/1

== system HF/Subsystem1/Speed2 ==
  Demux : Demux  Tag=STV Demux  Outputs=1
  FromWs : FromWorkspace  Tag=STV FromWs  VariableName=tuvar  SampleTime=0  SigBuilderData=DataTag2  VnvData=DataTag3
      SigBuilderData=|
      | common.afterFinalStr = 'Extrapolate'
      | common.sampleTime = 0
      | dataSet.timeRange = [0 10]
      | dataSet.name = '参考转速'
      | sbobj.Groups.Name = '参考转速'
      | sbobj.Groups.Signals.Name = 'Speed'
      | sbobj.Groups.Signals.XData = [0 0.5 1.5 2.5 10]
      | sbobj.Groups.Signals.YData = [10 100 100 1500 1500]
  Speed : Outport  Tag=STV Outport
  wires:
  Demux/1 -> Speed/1
  FromWs/1 -> Demux/1

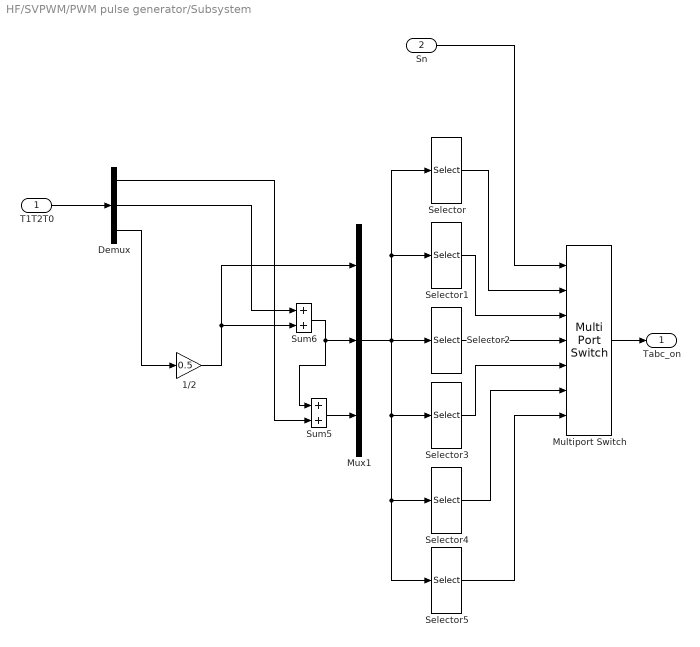
== system HF/SVPWM/PWM pulse generator/Subsystem ==
  T1T2T0 : Inport
  Sn : Inport  Port=2
  " 1/2" : Gain  Gain=0.5  SaturateOnIntegerOverflow=on  OutDataTypeStr=Inherit: Same as input  ParamDataTypeStr=Inherit: Same as input
  Demux : Demux  Outputs=3
  Multiport Switch : MultiPortSwitch  Inputs=6
  Mux1 : Mux  Inputs=3
  Selector : Selector  InputPortWidth=3  IndexOptions=Index vector (dialog)  Indices=[3 2 1]  OutputSizes=1
  Selector1 : Selector  InputPortWidth=3  IndexOptions=Index vector (dialog)  Indices=[2 3 1]  OutputSizes=1
  Selector2 : Selector  InputPortWidth=3  IndexOptions=Index vector (dialog)  Indices=[1 3 2]  OutputSizes=1
  Selector3 : Selector  InputPortWidth=3  IndexOptions=Index vector (dialog)  Indices=[1 2 3]  OutputSizes=1
  Selector4 : Selector  InputPortWidth=3  IndexOptions=Index vector (dialog)  Indices=[2 1 3]  OutputSizes=1
  Selector5 : Selector  InputPortWidth=3  IndexOptions=Index vector (dialog)  Indices=[3 1 2]  OutputSizes=1
  Sum5 : Sum  SaturateOnIntegerOverflow=on
  Sum6 : Sum  SaturateOnIntegerOverflow=on
  Tabc_on : Outport
  wires:
  Selector4/1 -> Multiport Switch/6
  Selector3/1 -> Multiport Switch/5
  Selector5/1 -> Multiport Switch/7
  Selector2/1 -> Multiport Switch/4
  Selector1/1 -> Multiport Switch/3
  Selector/1 -> Multiport Switch/2
  Sn/1 -> Multiport Switch/1
  Multiport Switch/1 -> Tabc_on/1
  Sum5/1 -> Mux1/3
  Sum6/1 -> Sum5/1, Mux1/2
  Mux1/1 -> Selector3/1, Selector4/1, Selector5/1, Selector2/1, Selector/1, Selector1/1
  " 1/2"/1 -> Sum6/2, Mux1/1
  T1T2T0/1 -> Demux/1
  Demux/2 -> Sum6/1
  Demux/3 -> " 1/2"/1
  Demux/1 -> Sum5/2

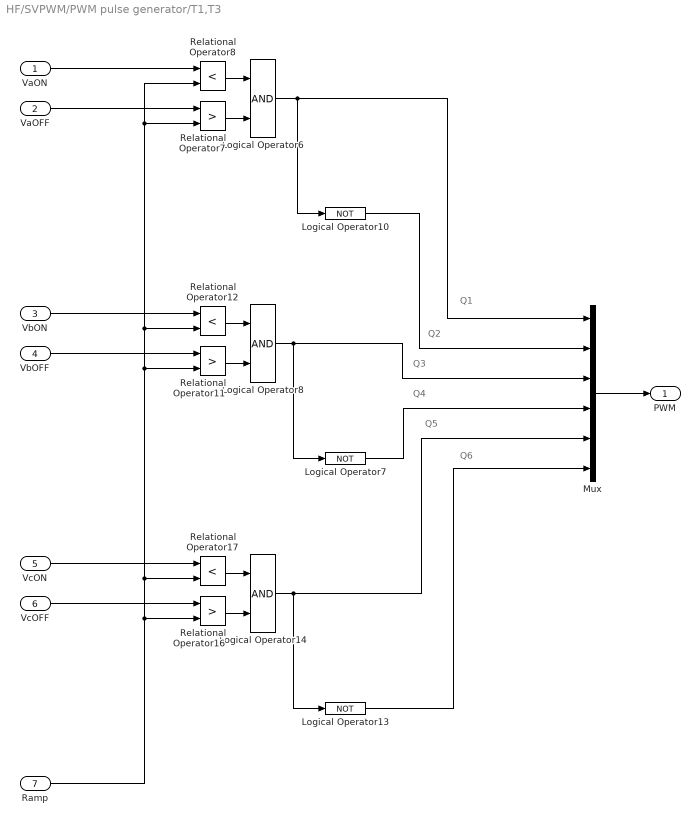
== system HF/SVPWM/PWM pulse generator/T1,T3 ==
  note: Q6
  note: Q5
  note: Q4
  note: Q3
  note: Q2
  note: Q1
  VaON : Inport
  VaOFF : Inport  Port=2
  VbON : Inport  Port=3
  VbOFF : Inport  Port=4
  VcON : Inport  Port=5
  VcOFF : Inport  Port=6
  Ramp : Inport  Port=7
  Logical Operator10 : Logic  Operator=NOT
  Logical Operator13 : Logic  Operator=NOT
  Logical Operator14 : Logic
  Logical Operator6 : Logic
  Logical Operator7 : Logic  Operator=NOT
  Logical Operator8 : Logic
  Mux : Mux  Inputs=6
  Relational Operator11 : RelationalOperator  Operator=>  RndMeth=Nearest  InputSameDT=on
  Relational Operator12 : RelationalOperator  Operator=<  RndMeth=Nearest  InputSameDT=on
  Relational Operator16 : RelationalOperator  Operator=>  RndMeth=Nearest  InputSameDT=on
  Relational Operator17 : RelationalOperator  Operator=<  RndMeth=Nearest  InputSameDT=on
  Relational Operator7 : RelationalOperator  Operator=>  RndMeth=Nearest  InputSameDT=on
  Relational Operator8 : RelationalOperator  Operator=<  RndMeth=Nearest  InputSameDT=on
  PWM : Outport
  wires:
  VcOFF/1 -> Relational Operator16/1
  VcON/1 -> Relational Operator17/1
  VbOFF/1 -> Relational Operator11/1
  VbON/1 -> Relational Operator12/1
  Mux/1 -> PWM/1
  Relational Operator8/1 -> Logical Operator6/1
  VaON/1 -> Relational Operator8/1
  Relational Operator7/1 -> Logical Operator6/2
  VaOFF/1 -> Relational Operator7/1
  Logical Operator6/1 -> Mux/1, Logical Operator10/1
  Relational Operator12/1 -> Logical Operator8/1
  Relational Operator11/1 -> Logical Operator8/2
  Logical Operator8/1 -> Mux/3, Logical Operator7/1
  Relational Operator17/1 -> Logical Operator14/1
  Relational Operator16/1 -> Logical Operator14/2
  Logical Operator14/1 -> Mux/5, Logical Operator13/1
  Ramp/1 -> Relational Operator16/2, Relational Operator17/2, Relational Operator11/2, Relational Operator7/2, Relational Operator8/2, Relational Operator12/2
  Logical Operator10/1 -> Mux/2
  Logical Operator7/1 -> Mux/4
  Logical Operator13/1 -> Mux/6
